simulink model "Power_electronics_ProjB_Q2"  (R2024b)
settings: Solver=VariableStepAuto  StartTime=0.0  StopTime=0.1  RelTol=1e-3
libraries: spsACCurrentSourceLib x3, spsRMSLib x2, spsACVoltageSourceLib x1, spsCurrentMeasurementLib x1, spsGroundLib x1, spsTHDLib x1, spsVoltageMeasurementLib x1, sps_lib x1
settings Model: Creator=MTMTAD006  LastModifiedBy=MTMTAD006

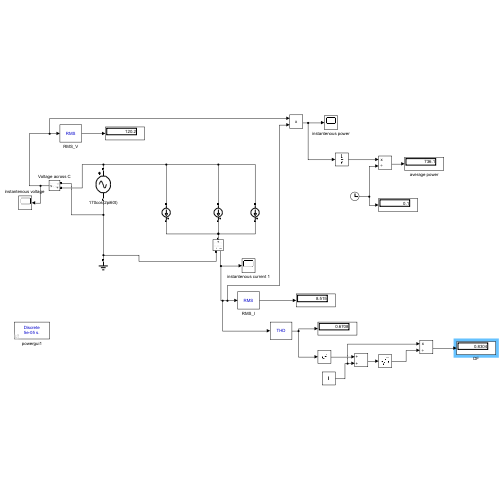
[thumbnail: Simulink's stored preview of the top-level diagram]
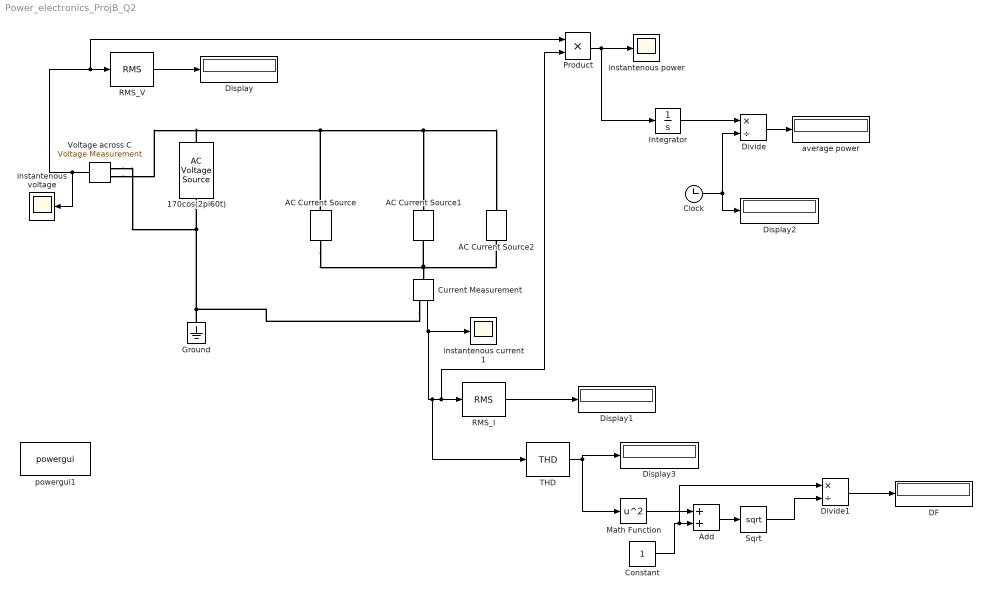
== system Power_electronics_ProjB_Q2 ==
  170cos(2pi60t) : spsACVoltageSourceLib/AC Voltage Source  Amplitude=170  Phase=90  Frequency=60  SampleTime=0  Measurements=None  BusType=swing  Pref=10e3  Qref=0  Qmin=-inf  Qmax=+inf
  AC Current Source : spsACCurrentSourceLib/AC Current Source  Amplitude=10  Phase=120  Frequency=60  SampleTime=0  Measurements=None
      settings: LibrarySourceBlock=sps_lib/Sources/AC Current Source
  AC Current Source1 : spsACCurrentSourceLib/AC Current Source  Amplitude=6  Phase=135  Frequency=120  SampleTime=0  Measurements=None
      settings: LibrarySourceBlock=sps_lib/Sources/AC Current Source
  AC Current Source2 : spsACCurrentSourceLib/AC Current Source  Amplitude=3  Phase=110  Frequency=240  SampleTime=0  Measurements=None
      settings: LibrarySourceBlock=sps_lib/Sources/AC Current Source
  Add : Sum
  Clock : Clock
  Constant : Constant
  Current Measurement : spsCurrentMeasurementLib/Current Measurement  PhasorSimulation=off  OutputType=Complex  PSBequivalent=0
  DF : Display
  Display{,1..3} (4 alike) : Display
  Divide : Product  Inputs=*/
  Divide1 : Product  Inputs=*/
  Ground : spsGroundLib/Ground  LConnTagsString=a
  Integrator : Integrator
  Math Function : Math  Operator=square
  Product : Product
  RMS_I : spsRMSLib/RMS  TrueRMS=on  Freq=60  RMSInit=120  Ts=0
  RMS_V : spsRMSLib/RMS  TrueRMS=on  Freq=60  RMSInit=120  Ts=0
  Sqrt : Sqrt
  THD : spsTHDLib/THD  Freq=60  Ts=0
  Voltage across C : spsVoltageMeasurementLib/Voltage Measurement  PhasorSimulation=off  OutputType=Complex  PSBequivalent=0
  average power : Display
  instantenous current 1 : Scope
  instantenous power : Scope
  "instantenous voltage " : Scope
  powergui1 : sps_lib/powergui  Priority=1  SimulationMode=Discrete  SampleTime=50e-6  frequency=60  Iterations=50  frequencyindice=60  Pbase=100e6  ErrMax=1e-4  UnitsV=kV  UnitsW=MW  buscounter=0  FunctionMessages=off  echomessages=off  EnableUseOfTLC=off  CurrentSourceSwitches=off  DisableSnubberDevices=off  DisableRonSwitches=off  DisableVfSwitches=off  DisplayEquations=off  AutomaticDiscreteSolvers=off  SolverType=Tustin/Backward Euler (TBE)  Interpol=off  ExternalGateDelay=off  methode=off  Ts=100  x0status=blocks  SPID=on  SwTol=0  HookPort=off  NonlinearTolerance=1e-4  nMaxIteration=100  ContinueOnMaxIteration=off  RestoreLinks=warning  ResistiveCurrentMeasurement=off  Frange=[0:2:500]  Ylog=off  Xlog=on  ShowGrid=off  save=off  variable=ZData  structure=0  ZoomFFT=off  StartTime=0.0  cycles=1  DisplayStyle=1  fundamental=60  FreqAxis=off  MaxFrequency=1000  frequencyindicesteady=1  RmsSteady=1  display=off
  wires:
  RMS_V/1 -> Display/1
  RMS_I/1 -> Display1/1
  Voltage across C/1 -> RMS_V/1, Product/1, "instantenous voltage "/1
  Current Measurement/1 -> THD/1, Product/2, RMS_I/1, instantenous current 1/1
  Product/1 -> instantenous power/1, Integrator/1
  Integrator/1 -> Divide/1
  Clock/1 -> Display2/1, Divide/2
  Divide/1 -> average power/1
  THD/1 -> Math Function/1, Display3/1
  Math Function/1 -> Add/1
  Constant/1 -> Divide1/1, Add/2
  Add/1 -> Sqrt/1
  Sqrt/1 -> Divide1/2
  Divide1/1 -> DF/1
  connections:
  AC Current Source/LConn1 -- Voltage across C/LConn1 -- 170cos(2pi60t)/RConn1 -- AC Current Source2/LConn1 -- AC Current Source1/LConn1
  AC Current Source/RConn1 -- Current Measurement/LConn1 -- AC Current Source1/RConn1 -- AC Current Source2/RConn1
  Ground/LConn1 -- Voltage across C/LConn2 -- 170cos(2pi60t)/LConn1 -- Current Measurement/RConn1
